simulink model "punkt3"  (R2015b)
settings: Solver=VariableStepAuto  StartTime=0.0  StopTime=15  RelTol=1e-3
settings Model: Creator=hohotulca  LastModifiedBy=hohotulca

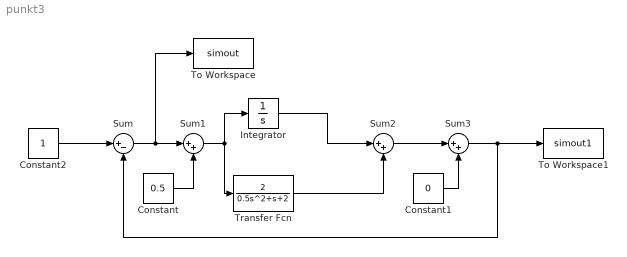
== system punkt3 ==
  Constant : Constant  Value=0.5
  Constant1 : Constant  Value=0
  Constant2 : Constant
  Integrator : Integrator
  Sum : Sum  Inputs=|+-
  Sum1 : Sum  Inputs=|++
  Sum2 : Sum  Inputs=|++
  Sum3 : Sum  Inputs=|++
  To Workspace : ToWorkspace  VariableName=simout  SaveFormat=Timeseries  SampleTime=-1
  To Workspace1 : ToWorkspace  VariableName=simout1  SaveFormat=Timeseries  SampleTime=-1
  Transfer Fcn : TransferFcn  Numerator=[ 2]  Denominator=[0.5 1 2]
  wires:
  Constant2/1 -> Sum/1
  Sum/1 -> To Workspace/1, Sum1/1
  Sum1/1 -> Transfer Fcn/1, Integrator/1
  Transfer Fcn/1 -> Sum2/2
  Integrator/1 -> Sum2/1
  Sum2/1 -> Sum3/1
  Sum3/1 -> To Workspace1/1, Sum/2
  Constant/1 -> Sum1/2
  Constant1/1 -> Sum3/2
